simulink model "hybrid_microgrid_model"  (R2024b)
settings: Solver=FixedStepDiscrete  StartTime=0.0  StopTime=8760  FixedStep=1  RelTol=1e-3
values from neighbouring files (symbols this model uses):
  Battery_Size_kWh = xopt(2)    [Project_run.m]
  DG_Size_kW = xopt(3)    [Project_run.m]
  PV_Size_kW = xopt(1)    [Project_run.m]
undefined symbols (not defined in the file or in its folder): DiscIntNeverNeededParam
settings Model: Creator=HP  LastModifiedBy=HP

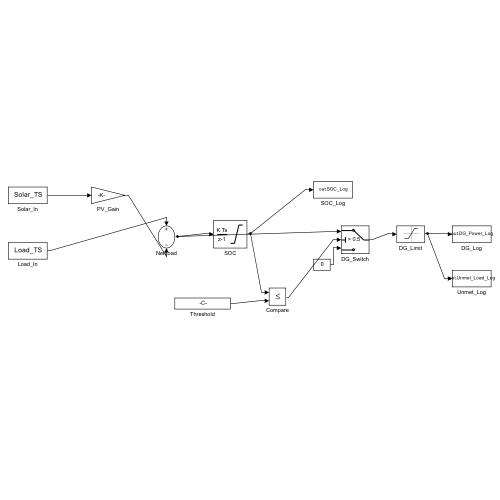
[thumbnail: Simulink's stored preview of the top-level diagram]
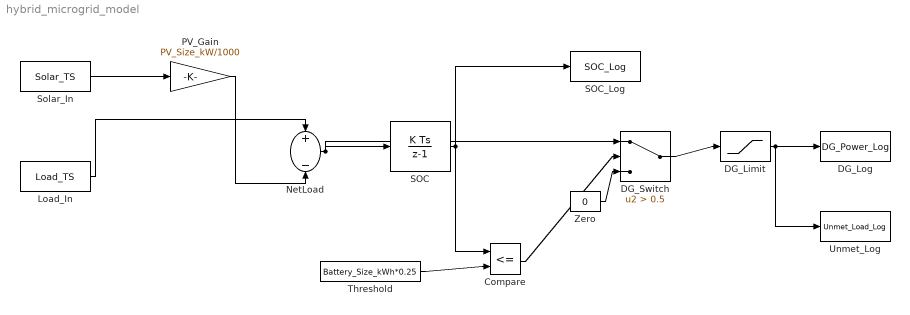
== system hybrid_microgrid_model ==
  Compare : RelationalOperator  Operator=<=  OutDataTypeStr=boolean  RndMeth=Simplest  InputSameDT=off
  DG_Limit : Saturate  UpperLimit=DG_Size_kW  LowerLimit=0
  DG_Log : ToWorkspace  VariableName=DG_Power_Log  SampleTime=-1
  DG_Switch : Switch  Criteria=u2 > Threshold  Threshold=0.5  SaturateOnIntegerOverflow=off  InputSameDT=off
  Load_In : FromWorkspace  VariableName=Load_TS
  NetLoad : Sum  Inputs=+-
  PV_Gain : Gain  Gain=PV_Size_kW/1000
  SOC : DiscreteIntegrator  InitialCondition=Battery_Size_kWh*0.8  SampleTime=-1  LimitOutput=on  UpperSaturationLimit=Battery_Size_kWh  LowerSaturationLimit=Battery_Size_kWh*0.2  ICPrevOutput=DiscIntNeverNeededParam  ICPrevScaledInput=DiscIntNeverNeededParam
  SOC_Log : ToWorkspace  VariableName=SOC_Log  SampleTime=-1
  Solar_In : FromWorkspace  VariableName=Solar_TS
  Threshold : Constant  Value=Battery_Size_kWh*0.25
  Unmet_Log : ToWorkspace  VariableName=Unmet_Load_Log  SampleTime=-1
  Zero : Constant  Value=0
  wires:
  Solar_In/1 -> PV_Gain/1
  Load_In/1 -> NetLoad/1
  PV_Gain/1 -> NetLoad/2
  NetLoad/1 -> SOC/1, DG_Switch/1
  SOC/1 -> SOC_Log/1, Compare/1
  Threshold/1 -> Compare/2
  Compare/1 -> DG_Switch/2
  Zero/1 -> DG_Switch/3
  DG_Switch/1 -> DG_Limit/1
  DG_Limit/1 -> DG_Log/1, Unmet_Log/1
